simulink subsystem "pam_rx"  (R2019b)
settings: Solver=VariableStepAuto  StartTime=0.0  StopTime=10.0  RelTol=1e-3
libraries: commutil2 x2, commdigbbndam3 x1
settings Model: Creator=yango  LastModifiedBy=yango

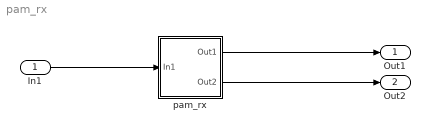
== system pam_rx ==
  In1 : Inport
  "pam_rx " : Subsystem
  Out1 : Outport  SignalName=symbol
  Out2 : Outport  Port=2  SignalName=bit
  wires:
  In1/1 -> "pam_rx "/1(In1)
  "pam_rx "/1(Out1) -> Out1/1
  "pam_rx "/2(Out2) -> Out2/1

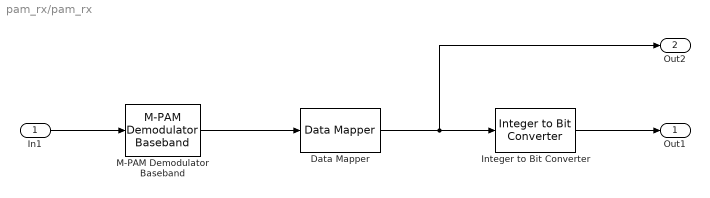
== system pam_rx/pam_rx  ==
  In1 : Inport
  Data Mapper : commutil2/Data Mapper  MapMode=Binary to Gray  M=4  MapVec=[0 1 3 2 7 6 4 5]
      settings: SourceProductName=Communications Toolbox  SourceProductBaseCode=CM
  Integer to Bit Converter : commutil2/Integer to Bit Converter  nbits=2  signedInputValues=Unsigned  bitOrder=MSB first  outDtype=Inherit via internal rule
      settings: SourceProductName=Communications Toolbox
  M-PAM Demodulator Baseband : commdigbbndam3/M-PAM Demodulator Baseband  M=4  OutType=Integer  Dec=Gray  PowType=Min. distance between symbols  MinDist=2  AvgPow=1  PeakPow=1  outDtype1=Inherit via internal rule  outDtype2=Inherit via internal rule  denormFactorWordLen=16  denormFactorDataTypeStr=Inherit: Same word length as input  denormFactorLastDataTypeStr=Inherit: Same word length as input  prodOutWordLen=16  prodOutRoundingMode=Floor  prodOutOverflowMode=Wrap  prodOutOvFlMode=off  prodOutOvFlModeLastStrValue=off  sumWordLen=16
      settings: SourceProductName=Communications Toolbox  SourceProductBaseCode=CM
  Out1 : Outport
  Out2 : Outport  Port=2
  wires:
  In1/1 -> M-PAM Demodulator Baseband/1
  M-PAM Demodulator Baseband/1 -> Data Mapper/1
  Integer to Bit Converter/1 -> Out1/1
  Data Mapper/1 -> Out2/1, Integer to Bit Converter/1
